simulink subsystem "noKalmanFilter"  (R2026a)
settings: Solver=VariableStepAuto
settings Model: Creator=maxhu  LastModifiedBy=maxhu

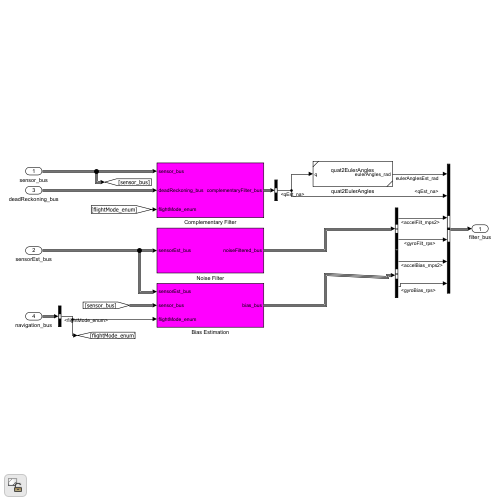
[thumbnail: Simulink's stored preview of the top-level diagram]
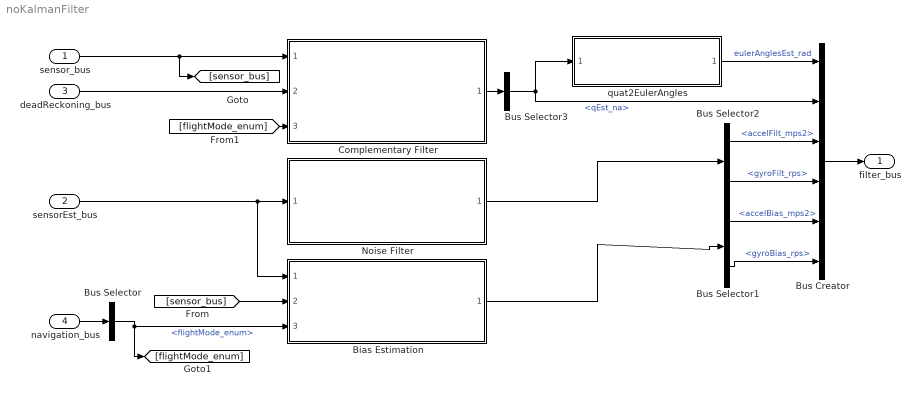
== system noKalmanFilter ==
  sensor_bus : Inport
  sensorEst_bus : Inport  Port=2
  deadReckoning_bus : Inport  Port=3
  navigation_bus : Inport  Port=4
  Bias Estimation : Subsystem  ReferencedSubsystem=biasEstimation
  Bus Creator : BusCreator  Inputs=6
  Bus Selector : BusSelector  OutputSignals=flightMode_enum
  Bus Selector1 : BusSelector  OutputSignals=accelBias_mps2,gyroBias_rps
  Bus Selector2 : BusSelector  OutputSignals=accelFilt_mps2,gyroFilt_rps
  Bus Selector3 : BusSelector  OutputSignals=qEst_na
  Complementary Filter : Subsystem  ReferencedSubsystem=compFilter
  Noise Filter : Subsystem  ReferencedSubsystem=noiseFilter
  quat2EulerAngles : Subsystem  ReferencedSubsystem=quat2EulerAngles
  filter_bus : Outport
  wires:
  navigation_bus/1 -> Bus Selector/1
  sensorEst_bus/1 -> Noise Filter/1, Bias Estimation/1
  Noise Filter/1 -> Bus Selector2/1
  Bus Selector/1 -> [flightMode_enum], Bias Estimation/3  "<flightMode_enum>"
  sensor_bus/1 -> Complementary Filter/1, [sensor_bus]
  Bias Estimation/1 -> Bus Selector1/1
  Bus Selector1/1 -> Bus Creator/5  "<accelBias_mps2>"
  Bus Selector1/2 -> Bus Creator/6  "<gyroBias_rps>"
  Bus Selector2/2 -> Bus Creator/4  "<gyroFilt_rps>"
  Bus Selector3/1 -> quat2EulerAngles/1, Bus Creator/2  "<qEst_na>"
  quat2EulerAngles/1 -> Bus Creator/1  "eulerAnglesEst_rad"
  Bus Selector2/1 -> Bus Creator/3  "<accelFilt_mps2>"
  Bus Creator/1 -> filter_bus/1
  [sensor_bus] -> Bias Estimation/2
  Complementary Filter/1 -> Bus Selector3/1
  [flightMode_enum] -> Complementary Filter/3
  deadReckoning_bus/1 -> Complementary Filter/2
